simulink model "PV_&_LV_FEEDER_MODEL"  (R2024b)
settings: Solver=ode23s  StartTime=0.0  StopTime=2.4  RelTol=1e-3
libraries: spsFirstOrderFilterLib x54, spsSeriesRLCBranchLib x12, spsThreePhaseVIMeasurementLib x9, spsIGBTDiodeLib x7, slpidlib x5, spsThreePhaseDynamicLoadLib x4, spsDistributedParametersLineLib x4, spsPower3phInstantaneousLib x4, simulink x3, spsThreePhaseSourceLib x2, spsThreePhaseTransformerTwoWindingsLib x2, spsabctodq0Lib x2
(part 2 of 3)

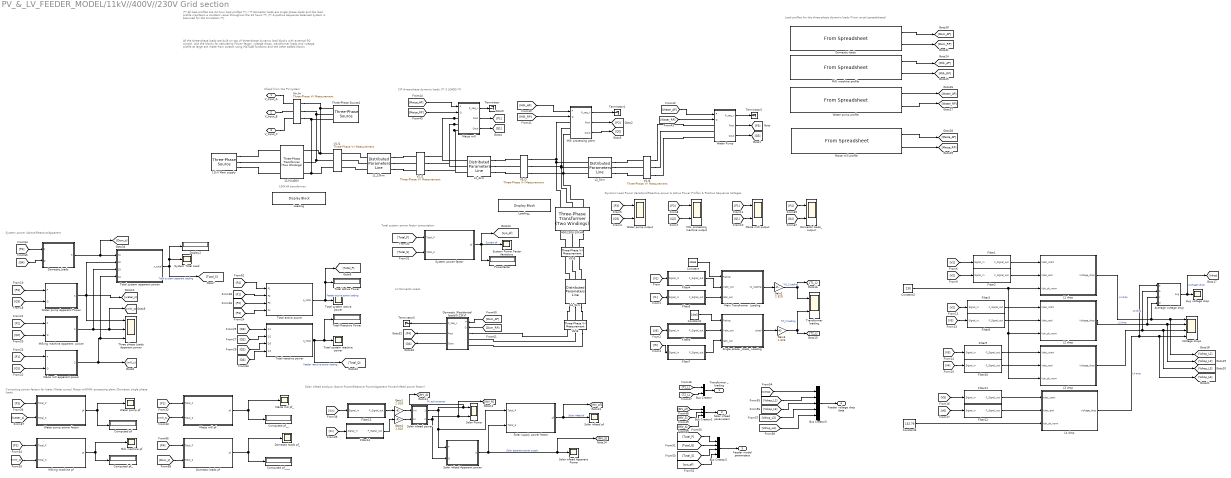
== system PV_&_LV_FEEDER_MODEL/11kV//400V//230V Grid section ==
  note: Load profiles for the three-phase dynamic loads (From excel spreadsheets)
  note: Total system power factor computation
  note: System power /Acitve/Reactive/Apparent
  note: 100kVA transformer
  note: Dynamic Load Power Variations(Reactive power & Active Power Profile) & Positive Sequence Voltages
  note: All the three-phase loads are built on top of three-phase dynamic load blocks with external PQ control.
      |
      | And the blocks for calculating Power factor, voltage drops, transfromer loads and voltage profile at large are made from scratch using MATLAB functions and the other added blocks
  note: Infeed from the PV system
  note: LV Domestic Loads
  note: CIP three-phase dynamic loads /** 3 LOADS **/
  note: /** All load profiles are 24 hour load profiles **/
      |
      | / ** Domestic loads are single phase loads and the load profile maintains a constant value throughout the 24 hours **/
      |
      | /** A postive sequence balanced system is assumed for the simulation **/
  note: Solar infeed analysis (Active Power/Reactive Power/Apparent Power/Infeed power factor)
  note: Computing power factors for loads /Water pump/ Maize mill/Milk processing plant /Domestic single phase loads
  11kV Main supply : spsThreePhaseSourceLib/Three-Phase Source  InternalConnection=Yg  VoltagePhases=off  Voltage=11e3  PhaseAngle=0  Voltage_phases=[25e3 25e3 25e3]/sqrt(3)  PhaseAngles_phases=[0 -120 +120]  Frequency=50  NonIdealSource=on  SpecifyImpedance=off  Resistance=0.8929  Inductance=16.58e-3  ShortCircuitLevel=100e6  BaseVoltage=25e3  XRratio=7  BusType=swing  Pref=10e3  Qref=0  Prefabc=[10e3, 10e3, 10e3]  Qrefabc=[0, 0, 0]  Qmin=-inf  Qmax=inf
  "11kV/400V " : spsThreePhaseTransformerTwoWindingsLib/Three-Phase Transformer (Two Windings)  Winding1Connection=Yg  Winding2Connection=Yg  CoreType=Three single-phase transformers  SetSaturation=off  Hysteresis=off  DataFile='hysteresis'  SetInitialFlux=off  Measurements=None  UNITS=pu  NominalPower=[ 100e3 , 50 ]  Winding1=[ 11e3 , 0.002 , 0.08 ]  Winding2=[ 400 , 0.002 , 0.08 ]  Rm=500  Lm=500  L0=0.5  Saturation=[ 0,0 ; 0.0024,1.2 ; 1.0,1.52 ]  InitialFluxes=[ 0.8 , -0.8 , 0.7 ]  BreakLoop=off  DiscreteSolver=Trapezoidal iterative  DataType=off  TransfoNumber=1
  "400/230V-10kVA " : spsThreePhaseTransformerTwoWindingsLib/Three-Phase Transformer (Two Windings)  Winding1Connection=Yg  Winding2Connection=Yg  CoreType=Three single-phase transformers  SetSaturation=off  Hysteresis=off  DataFile='hysteresis'  SetInitialFlux=off  Measurements=None  UNITS=pu  NominalPower=[ 10e3 , 50 ]  Winding1=[ 400 , 0.002 , 0.08 ]  Winding2=[ 230 , 0.002 , 0.08 ]  Rm=500  Lm=500  L0=0.5  Saturation=[ 0,0 ; 0.0024,1.2 ; 1.0,1.52 ]  InitialFluxes=[ 0.8 , -0.8 , 0.7 ]  BreakLoop=off  DiscreteSolver=Trapezoidal iterative  DataType=off  TransfoNumber=1
  Average voltage drop : MATLAB Function  TreatAsAtomicUnit=on
  Avg voltage drop : Scope
  Bus Creator : BusCreator  Inputs=2
  Bus Creator1 : BusCreator  Inputs=3
  Bus Creator2 : BusCreator  Inputs=4
  Bus Creator3 : BusCreator  Inputs=5
  Computed pf : Display
  Computed pf_ : Display
  Computed pf__ : Display
  Computed pf____ : Display
  Constant : Constant  Value=100e3
  Constant1 : Constant  Value=10e3
  Constant2 : Constant  Value=230
  Constant3 : Constant  Value=132.79
  Display2 : Display
  Domestic /Residential loads(0.23kV) : Subsystem
  Domestic loads : FromSpreadsheet  FileName=C:\Users\Baymax\Desktop\Mr.Usamah\Profiles\granular\h_pf\Domestic_loads.xlsx  SheetName=profile  Range=A2:C2002
  Domestic loads pf : MATLAB Function  TreatAsAtomicUnit=on
  Domestic loads pf_ : Scope
  Domestic loads_output : Scope  NumInputPorts=2
  Domestic_loads : MATLAB Function  TreatAsAtomicUnit=on
  Filter1 : Subsystem
  Filter10 : Subsystem
  Filter11 : Subsystem
  Filter12 : Subsystem
  Filter13 : Subsystem
  Filter14 : Subsystem
  Filter2 : Subsystem
  Filter3 : Subsystem
  Filter4 : Subsystem
  Filter5 : Subsystem
  Filter6 : Subsystem
  Filter7 : Subsystem
  Filter8 : Subsystem
  Filter9 : Subsystem
  Gain{1..4} (4 alike) : Gain  Gain=2.828
  L1 drop : Subsystem
  L1_10km : spsDistributedParametersLineLib/Distributed Parameters Line  Phases=3  Length=10  Frequency=50  Resistance=[0.01273 0.3864]  Inductance="[0.9337e-3  4.1264e-3]"  Capacitance=[12.74e-9 7.751e-9]  x1=[-5.7e-05 -1.52676771420257e-15 0 0;-5.6e-05 -1.49998510389932e-15 0 0;-5.5e-05 -1.47320234555348e-15 0 0;-5.4e-05 -1.44641944180839e-15 0 0;-5.3e-05 -1.41963639530743e-15 0 0;-5.2e-05 -1.39285320869397e-15 0 0;-5.1e-05 -1.36606988461142e-15 0 0;-5e-05 -1.33928642570317e-15 0 0;-4.9e-05 -1.31250283461264e-15 0 0;-4.8e-05 -1.28571911398329e-15 0 0;-4.7e-05 -1.25893526645854e-15 0 0;-4.6e-05 -1.23215129468186e-15 0 0;-4.5e-05 -1.20536720129673e-15 0 0;-4.4e-05 -1.17858298894662e-15 0 0;-4.3e-05 -1.15179866027504e-15 0 0;-4.2e-05 -1.12501421792548e-15 0 0;-4.1e-05 -1.09822966454148e-15 0 0;-4e-05 -1.07144500276655e-15 0 0;-3.9e-05 -1.04466023524424e-15 0 0;-3.8e-05 -1.01787536461809e-15 0 0;-3.7e-05 -9.91090393531678e-16 0 0;-3.6e-05 -9.64305324628563e-16 0 0;-3.5e-05 -9.37520160552329e-16 196.179007943669 -348.588291315468;-3.4e-05 -9.10734903946564e-16 196.288510502334 -348.526642661325;-3.3e-05 -8.83949557454868e-16 196.3979936881 -348.464959608981;-3.2e-05 -8.57164123720848e-16 196.507457490161 -348.403242164525;-3.1e-05 -8.30378605388121e-16 196.616901897713 -348.341490334047;-3e-05 -8.03593005100311e-16 196.726326899956 -348.279704123642;-2.9e-05 -7.76807325501051e-16 196.835732486088 -348.217883539409;-2.8e-05 -7.50021569233982e-16 196.945118645312 -348.156028587448;-2.7e-05 -7.23235738942752e-16 197.054485366832 -348.094139273865;-2.6e-05 -6.96449837271016e-16 197.163832639854 -348.032215604768;-2.5e-05 -6.69663866862436e-16 197.273160453586 -347.970257586268;-2.4e-05 -6.42877830360683e-16 197.382468797238 -347.90826522448;-2.3e-05 -6.16091730409431e-16 197.491757660021 -347.846238525524;-2.2e-05 -5.89305569652364e-16 197.601027031149 -347.78417749552;-2.1e-05 -5.62519350733168e-16 197.710276899837 -347.722082140594;-2e-05 -5.35733076295539e-16 197.819507255304 -347.659952466874;-1.9e-05 -5.08946748983174e-16 197.928718086768 -347.597788480492;-1.8e-05 -4.82160371439779e-16 198.03790938345 -347.535590187584;-1.7e-05 -4.55373946309064e-16 198.147081134575 -347.473357594289;-1.6e-05 -4.28587476234741e-16 198.256233329366 -347.411090706748;-1.5e-05 -4.01800963860531e-16 198.365365957052 -347.348789531107;-1.4e-05 -3.75014411830155e-16 198.474479006861 -347.286454073514;-1.3e-05 -3.48227822787341e-16 198.583572468024 -347.224084340123;-1.2e-05 -3.21441199375819e-16 198.692646329775 -347.161680337089;-1.1e-05 -2.94654544239322e-16 198.801700581347 -347.09924207057;-1e-05 -2.67867860021587e-16 198.910735211978 -347.03676954673;-9e-06 -2.41081149366355e-16 199.019750210907 -346.974262771734;-8e-06 -2.14294414917367e-16 199.128745567374 -346.911721751751;-7e-06 -1.87507659318368e-16 199.237721270622 -346.849146492953;-6e-06 -1.60720885213105e-16 199.346677309894 -346.786537001518;-5e-06 -1.33934095245327e-16 199.455613674439 -346.723893283623;-4e-06 -1.07147292058783e-16 199.564530353504 -346.661215345452;-3e-06 -8.03604782972257e-17 199.673427336339 -346.59850319319;-2e-06 -5.35736566044071e-17 199.782304612197 -346.535756833028;-1e-06 -2.67868296240806e-17 199.891162170332 -346.472976271158]  x2=[-5.7e-05 -2.62897177572208e-12 0 0;-5.6e-05 -2.62972765843218e-12 0 0;-5.5e-05 -2.63048328159856e-12 0 0;-5.4e-05 -2.63123864514666e-12 0 0;-5.3e-05 -2.63199374900191e-12 0 0;-5.2e-05 -2.63274859308979e-12 0 0;-5.1e-05 -2.6335031773358e-12 0 0;-5e-05 -2.63425750166547e-12 0 0;-4.9e-05 -2.63501156600435e-12 0 0;-4.8e-05 -2.63576537027801e-12 0 0;-4.7e-05 -2.63651891441206e-12 0 0;-4.6e-05 -2.63727219833213e-12 0 0;-4.5e-05 -2.63802522196386e-12 0 0;-4.4e-05 -2.63877798523294e-12 0 0;-4.3e-05 -2.63953048806508e-12 0 0;-4.2e-05 -2.640282730386e-12 0 0;-4.1e-05 -2.64103471212147e-12 0 0;-4e-05 -2.64178643319725e-12 0 0;-3.9e-05 -2.64253789353917e-12 0 0;-3.8e-05 -2.64328909307306e-12 0 0;-3.7e-05 -2.64404003172477e-12 0 0;-3.6e-05 -2.64479070942019e-12 0 0;-3.5e-05 -2.64554112608523e-12 132.127149459759 -329.646500354157;-3.4e-05 -2.64629128164583e-12 132.230307052903 -329.60328299373;-3.3e-05 -2.64704117602796e-12 132.33345159544 -329.560033102763;-3.2e-05 -2.64779080915759e-12 132.436583077188 -329.516750685525;-3.1e-05 -2.64854018096075e-12 132.539701487969 -329.473435746288;-3e-05 -2.64928929136347e-12 132.642806817607 -329.430088289326;-2.9e-05 -2.65003814029182e-12 132.745899055924 -329.386708318918;-2.8e-05 -2.65078672767189e-12 132.848978192746 -329.343295839345;-2.7e-05 -2.6515350534298e-12 132.9520442179 -329.299850854891;-2.6e-05 -2.65228311749169e-12 133.055097121213 -329.256373369846;-2.5e-05 -2.65303091978374e-12 133.158136892514 -329.212863388499;-2.4e-05 -2.65377846023213e-12 133.261163521634 -329.169320915145;-2.3e-05 -2.65452573876308e-12 133.364176998405 -329.125745954082;-2.2e-05 -2.65527275530285e-12 133.467177312659 -329.08213850961;-2.1e-05 -2.6560195097777e-12 133.570164454231 -329.038498586033;-2e-05 -2.65676600211394e-12 133.673138412956 -328.994826187658;-1.9e-05 -2.65751223223789e-12 133.776099178671 -328.951121318796;-1.8e-05 -2.65825820007589e-12 133.879046741214 -328.907383983759;-1.7e-05 -2.65900390555433e-12 133.981981090426 -328.863614186865;-1.6e-05 -2.6597493485996e-12 134.084902216146 -328.819811932434;-1.5e-05 -2.66049452913813e-12 134.187810108216 -328.775977224788;-1.4e-05 -2.66123944709639e-12 134.290704756481 -328.732110068254;-1.3e-05 -2.66198410240084e-12 134.393586150785 -328.688210467162;-1.2e-05 -2.66272849497799e-12 134.496454280973 -328.644278425844;-1.1e-05 -2.66347262475438e-12 134.599309136893 -328.600313948636;-1e-05 -2.66421649165655e-12 134.702150708395 -328.556317039877;-9e-06 -2.6649600956111e-12 134.804978985327 -328.51228770391;-8e-06 -2.66570343654463e-12 134.907793957541 -328.468225945079;-7e-06 -2.66644651438379e-12 135.010595614889 -328.424131767735;-6e-06 -2.66718932905522e-12 135.113383947226 -328.380005176228;-5e-06 -2.66793188048562e-12 135.216158944407 -328.335846174914;-4e-06 -2.66867416860169e-12 135.318920596287 -328.291654768151;-3e-06 -2.66941619333019e-12 135.421668892726 -328.247430960301;-2e-06 -2.67015795459787e-12 135.524403823582 -328.203174755729;-1e-06 -2.67089945233153e-12 135.627125378715 -328.158886158801]  x3=[-5.7e-05 1.17698290725369e-13 0 0;-5.6e-05 1.1762296132752e-13 0 0;-5.5e-05 1.1754762032075e-13 0 0;-5.4e-05 1.17472267712495e-13 0 0;-5.3e-05 1.17396903510192e-13 0 0;-5.2e-05 1.17321527721279e-13 0 0;-5.1e-05 1.17246140353195e-13 0 0;-5e-05 1.17170741413382e-13 0 0;-4.9e-05 1.17095330909279e-13 0 0;-4.8e-05 1.17019908848331e-13 0 0;-4.7e-05 1.16944475237981e-13 0 0;-4.6e-05 1.16869030085674e-13 0 0;-4.5e-05 1.16793573398857e-13 0 0;-4.4e-05 1.16718105184975e-13 0 0;-4.3e-05 1.16642625451479e-13 0 0;-4.2e-05 1.16567134205817e-13 0 0;-4.1e-05 1.1649163145544e-13 0 0;-4e-05 1.16416117207799e-13 0 0;-3.9e-05 1.16340591470349e-13 0 0;-3.8e-05 1.16265054250543e-13 0 0;-3.7e-05 1.16189505555836e-13 0 0;-3.6e-05 1.16113945393684e-13 0 0;-3.5e-05 1.16038373771546e-13 6.64607990253194 18.9464899277629;-3.4e-05 1.15962790696879e-13 6.63954583439883 18.948466711769;-3.3e-05 1.15887196177143e-13 6.63301111096882 18.9504416256364;-3.2e-05 1.158115902198e-13 6.62647573288685 18.9524146691702;-3.1e-05 1.15735972832311e-13 6.61993970079795 18.9543858421757;-3e-05 1.1566034402214e-13 6.6134030153472 18.9563551444583;-2.9e-05 1.1558470379675e-13 6.60686567717974 18.9583225758237;-2.8e-05 1.15509052163607e-13 6.60032768694077 18.9602881360776;-2.7e-05 1.15433389130178e-13 6.59378904527558 18.9622518250261;-2.6e-05 1.1535771470393e-13 6.58724975282951 18.9642136424754;-2.5e-05 1.15282028892332e-13 6.58070981024794 18.9661735882318;-2.4e-05 1.15206331702854e-13 6.57416921817636 18.968131662102;-2.3e-05 1.15130623142967e-13 6.56762797726028 18.9700878638926;-2.2e-05 1.15054903220143e-13 6.56108608814531 18.9720421934106;-2.1e-05 1.14979171941855e-13 6.55454355147711 18.9739946504631;-2e-05 1.14903429315578e-13 6.54800036790139 18.9759452348574;-1.9e-05 1.14827675348787e-13 6.54145653806395 18.977893946401;-1.8e-05 1.14751910048959e-13 6.53491206261062 18.9798407849015;-1.7e-05 1.14676133423572e-13 6.52836694218734 18.9817857501669;-1.6e-05 1.14600345480103e-13 6.52182117744007 18.9837288420051;-1.5e-05 1.14524546226035e-13 6.51527476901485 18.9856700602244;-1.4e-05 1.14448735668846e-13 6.5087277175578 18.9876094046332;-1.3e-05 1.1437291381602e-13 6.50218002371507 18.9895468750401;-1.2e-05 1.14297080675041e-13 6.4956316881329 18.9914824712538;-1.1e-05 1.14221236253391e-13 6.48908271145759 18.9934161930834;-1e-05 1.14145380558558e-13 6.48253309433549 18.9953480403379;-9e-06 1.14069513598027e-13 6.47598283741302 18.9972780128267;-8e-06 1.13993635379286e-13 6.46943194133667 18.9992061103594;-7e-06 1.13917745909825e-13 6.46288040675299 19.0011323327456;-6e-06 1.13841845197133e-13 6.45632823430858 19.0030566797952;-5e-06 1.13765933248701e-13 6.44977542465012 19.0049791513184;-4e-06 1.13690010072022e-13 6.44322197842435 19.0068997471252;-3e-06 1.13614075674589e-13 6.43666789627806 19.0088184670263;-2e-06 1.13538130063896e-13 6.43011317885812 19.0107353108322;-1e-06 1.13462173247438e-13 6.42355782681145 19.0126502783538]  x4=[-5.7e-05 -1.21011045818771e-13 0 0;-5.6e-05 -1.20939770771355e-13 0 0;-5.5e-05 -1.20868483787662e-13 0 0;-5.4e-05 -1.20797184874728e-13 0 0;-5.3e-05 -1.2072587403959e-13 0 0;-5.2e-05 -1.20654551289286e-13 0 0;-5.1e-05 -1.20583216630855e-13 0 0;-5e-05 -1.20511870071338e-13 0 0;-4.9e-05 -1.20440511617776e-13 0 0;-4.8e-05 -1.20369141277212e-13 0 0;-4.7e-05 -1.2029775905669e-13 0 0;-4.6e-05 -1.20226364963256e-13 0 0;-4.5e-05 -1.20154959003954e-13 0 0;-4.4e-05 -1.20083541185834e-13 0 0;-4.3e-05 -1.20012111515944e-13 0 0;-4.2e-05 -1.19940670001333e-13 0 0;-4.1e-05 -1.19869216649052e-13 0 0;-4e-05 -1.19797751466154e-13 0 0;-3.9e-05 -1.19726274459692e-13 0 0;-3.8e-05 -1.1965478563672e-13 0 0;-3.7e-05 -1.19583285004294e-13 0 0;-3.6e-05 -1.19511772569472e-13 0 0;-3.5e-05 -1.1944024833931e-13 -5.44733327904661 -21.4575907170846;-3.4e-05 -1.19368712320869e-13 -5.44001188573569 -21.4591845394917;-3.3e-05 -1.19297164521207e-13 -5.43268995551713 -21.4607762439623;-3.2e-05 -1.19225604947388e-13 -5.42536748911357 -21.4623658303391;-3.1e-05 -1.19154033606473e-13 -5.4180444872477 -21.4639532984654;-3e-05 -1.19082450505527e-13 -5.41072095064228 -21.4655386481844;-2.9e-05 -1.19010855651614e-13 -5.40339688002011 -21.4671218793397;-2.8e-05 -1.189392490518e-13 -5.39607227610405 -21.4687029917749;-2.7e-05 -1.18867630713153e-13 -5.38874713961701 -21.4702819853342;-2.6e-05 -1.18796000642742e-13 -5.38142147128195 -21.4718588598616;-2.5e-05 -1.18724358847635e-13 -5.37409527182188 -21.4734336152014;-2.4e-05 -1.18652705334903e-13 -5.36676854195987 -21.4750062511983;-2.3e-05 -1.18581040111619e-13 -5.35944128241904 -21.4765767676971;-2.2e-05 -1.18509363184856e-13 -5.35211349392256 -21.4781451645427;-2.1e-05 -1.18437674561687e-13 -5.34478517719366 -21.4797114415804;-2e-05 -1.18365974249189e-13 -5.33745633295561 -21.4812755986556;-1.9e-05 -1.18294262254437e-13 -5.33012696193174 -21.4828376356138;-1.8e-05 -1.1822253858451e-13 -5.32279706484543 -21.484397552301;-1.7e-05 -1.18150803246486e-13 -5.31546664242011 -21.4859553485632;-1.6e-05 -1.18079056247445e-13 -5.30813569537926 -21.4875110242466;-1.5e-05 -1.18007297594468e-13 -5.30080422444643 -21.4890645791976;-1.4e-05 -1.17935527294638e-13 -5.29347223034519 -21.490616013263;-1.3e-05 -1.17863745355039e-13 -5.28613971379918 -21.4921653262897;-1.2e-05 -1.17791951782754e-13 -5.27880667553211 -21.4937125181247;-1.1e-05 -1.17720146584869e-13 -5.2714731162677 -21.4952575886152;-1e-05 -1.17648329768472e-13 -5.26413903672975 -21.496800537609;-9e-06 -1.1757650134065e-13 -5.25680443764211 -21.4983413649535;-8e-06 -1.17504661308492e-13 -5.24946931972867 -21.4998800704969;-7e-06 -1.1743280967909e-13 -5.24213368371339 -21.5014166540871;-6e-06 -1.17360946459533e-13 -5.23479753032024 -21.5029511155726;-5e-06 -1.17289071656916e-13 -5.2274608602733 -21.5044834548019;-4e-06 -1.17217185278332e-13 -5.22012367429665 -21.5060136716238;-3e-06 -1.17145287330875e-13 -5.21278597311445 -21.5075417658872;-2e-06 -1.17073377821642e-13 -5.2054477574509 -21.5090677374414;-1e-06 -1.17001456757729e-13 -5.19810902803026 -21.5105915861357]  x5=5.65541566995743e-05  V1=ones(3,3)  V2=ones(3,3)  I1=ones(3,3)  I2=ones(3,3)  nHarmo=1  Measurements=None  Decoupling=off  VsMag0=0  VrMag0=0  VsAngle0=0  VrAngle0=0  IsMag0=0  IrMag0=0  IsAngle0=0  IrAngle0=0
      settings: LibrarySourceBlock=sps_lib/Power Grid Elements/Distributed Parameters Line
  L2 drop : Subsystem
  L2_3km : spsDistributedParametersLineLib/Distributed Parameters Line  Phases=3  Length=3  Frequency=50  Resistance=[0.01273 0.3864]  Inductance="[0.9337e-3  4.1264e-3]"  Capacitance=[12.74e-9 7.751e-9]  x1=[-1.7e-05 -2.65900390555433e-12 0 0;-1.6e-05 -2.6597493485996e-12 0 0;-1.5e-05 -2.66049452913813e-12 0 0;-1.4e-05 -2.66123944709639e-12 0 0;-1.3e-05 -2.66198410240084e-12 0 0;-1.2e-05 -2.66272849497799e-12 0 0;-1.1e-05 -2.66347262475438e-12 134.599309136893 -328.600313948636;-1e-05 -2.66421649165655e-12 134.702150708395 -328.556317039877;-9e-06 -2.6649600956111e-12 134.804978985327 -328.51228770391;-8e-06 -2.66570343654463e-12 134.907793957541 -328.468225945079;-7e-06 -2.66644651438379e-12 135.010595614889 -328.424131767735;-6e-06 -2.66718932905522e-12 135.113383947226 -328.380005176228;-5e-06 -2.66793188048562e-12 135.216158944407 -328.335846174914;-4e-06 -2.66867416860169e-12 135.318920596287 -328.291654768151;-3e-06 -2.66941619333019e-12 135.421668892726 -328.247430960301;-2e-06 -2.67015795459787e-12 135.524403823582 -328.203174755729;-1e-06 -2.67089945233153e-12 135.627125378715 -328.158886158801]  x2=[-1.7e-05 -1.06786625029648e-12 0 0;-1.6e-05 -1.06858231496139e-12 0 0;-1.5e-05 -1.06929827416146e-12 0 0;-1.4e-05 -1.07001412782602e-12 0 0;-1.3e-05 -1.07072987588442e-12 0 0;-1.2e-05 -1.07144551826601e-12 0 0;-1.1e-05 -1.07216105490018e-12 117.837536827924 -323.773646079117;-1e-05 -1.07287648571629e-12 117.938747506776 -323.73440678193;-9e-06 -1.07359181064373e-12 118.039946545541 -323.695135533439;-8e-06 -1.07430702961191e-12 118.14113393423 -323.655832337518;-7e-06 -1.07502214255024e-12 118.242309662856 -323.616497198048;-6e-06 -1.07573714938814e-12 118.343473721435 -323.57713011891;-5e-06 -1.07645205005503e-12 118.44462609998 -323.537731103989;-4e-06 -1.07716684448037e-12 118.54576678851 -323.498300157174;-3e-06 -1.0778815325936e-12 118.646895777042 -323.458837282357;-2e-06 -1.07859611432419e-12 118.748013055595 -323.419342483433;-1e-06 -1.07931058960162e-12 118.849118614188 -323.379815764299]  x3=[-1.7e-05 6.00604604613741e-14 0 0;-1.6e-05 6.01818414409508e-14 0 0;-1.5e-05 6.0303216480818e-14 0 0;-1.4e-05 6.04245855689962e-14 0 0;-1.3e-05 6.0545948693507e-14 0 0;-1.2e-05 6.06673058423722e-14 0 0;-1.1e-05 6.07886570036144e-14 5.56089804964976 16.1978590482491;-1e-05 6.09100021652566e-14 5.5552252459904 16.199505686642;-9e-06 6.10313413153226e-14 5.5495518940523 16.2011507262079;-8e-06 6.11526744418368e-14 5.54387799439538 16.2027941667843;-7e-06 6.12740015328239e-14 5.53820354757964 16.204436008209;-6e-06 6.13953225763096e-14 5.53252855416512 16.20607625032;-5e-06 6.15166375603198e-14 5.52685301471193 16.2077148929554;-4e-06 6.16379464728813e-14 5.52117692978021 16.2093519359535;-3e-06 6.17592493020214e-14 5.51550029993018 16.2109873791527;-2e-06 6.18805460357679e-14 5.50982312572209 16.2126212223915;-1e-06 6.20018366621494e-14 5.50414540771625 16.2142534655088]  x4=[-1.7e-05 -6.87075593118103e-14 0 0;-1.6e-05 -6.88423373437948e-14 0 0;-1.5e-05 -6.89771085813131e-14 0 0;-1.4e-05 -6.91118730110636e-14 0 0;-1.3e-05 -6.92466306197458e-14 0 0;-1.2e-05 -6.93813813940595e-14 0 0;-1.1e-05 -6.95161253207054e-14 -4.63242844236993 -18.6089754457082;-1e-05 -6.96508623863848e-14 -4.62600150068479 -18.6103158835768;-9e-06 -6.97855925777997e-14 -4.6195741024316 -18.6116544846809;-8e-06 -6.99203158816527e-14 -4.61314624824473 -18.6129912488883;-7e-06 -7.00550322846471e-14 -4.60671793875858 -18.6143261760672;-6e-06 -7.01897417734871e-14 -4.60028917460759 -18.6156592660857;-5e-06 -7.03244443348774e-14 -4.59385995642626 -18.6169905188123;-4e-06 -7.04591399555232e-14 -4.58743028484914 -18.6183199341155;-3e-06 -7.05938286221307e-14 -4.58100016051079 -18.6196475118643;-2e-06 -7.07285103214066e-14 -4.57456958404586 -18.6209732519275;-1e-06 -7.08631850400584e-14 -4.56813855608901 -18.6222971541744]  x5=1.69662470098723e-05  V1=ones(3,3)  V2=ones(3,3)  I1=ones(3,3)  I2=ones(3,3)  nHarmo=1  Measurements=None  Decoupling=off  VsMag0=0  VrMag0=0  VsAngle0=0  VrAngle0=0  IsMag0=0  IrMag0=0  IsAngle0=0  IrAngle0=0
      settings: LibrarySourceBlock=sps_lib/Power Grid Elements/Distributed Parameters Line
  L3 drop : Subsystem
  L3_5km : spsDistributedParametersLineLib/Distributed Parameters Line  Phases=3  Length=5  Frequency=50  Resistance=[0.01273 0.3864]  Inductance="[0.9337e-3  4.1264e-3]"  Capacitance=[12.74e-9 7.751e-9]  x1=[-2.9e-05 -1.05926527379479e-12 0 0;-2.8e-05 -1.05998259852241e-12 0 0;-2.7e-05 -1.06069981863395e-12 0 0;-2.6e-05 -1.06141693405861e-12 0 0;-2.5e-05 -1.06213394472562e-12 0 0;-2.4e-05 -1.06285085056421e-12 0 0;-2.3e-05 -1.06356765150363e-12 0 0;-2.2e-05 -1.06428434747313e-12 0 0;-2.1e-05 -1.06500093840198e-12 0 0;-2e-05 -1.06571742421944e-12 0 0;-1.9e-05 -1.06643380485482e-12 0 0;-1.8e-05 -1.06715008023739e-12 117.128736992729 -324.047426197968;-1.7e-05 -1.06786625029648e-12 117.230028872437 -324.008410668177;-1.6e-05 -1.06858231496139e-12 117.331309182004 -323.969363160038;-1.5e-05 -1.06929827416146e-12 117.432577911436 -323.930283677405;-1.4e-05 -1.07001412782602e-12 117.533835050737 -323.891172224135;-1.3e-05 -1.07072987588442e-12 117.635080589913 -323.852028804087;-1.2e-05 -1.07144551826601e-12 117.736314518973 -323.812853421126;-1.1e-05 -1.07216105490018e-12 117.837536827924 -323.773646079117;-1e-05 -1.07287648571629e-12 117.938747506776 -323.73440678193;-9e-06 -1.07359181064373e-12 118.039946545541 -323.695135533439;-8e-06 -1.07430702961191e-12 118.14113393423 -323.655832337518;-7e-06 -1.07502214255024e-12 118.242309662856 -323.616497198048;-6e-06 -1.07573714938814e-12 118.343473721435 -323.57713011891;-5e-06 -1.07645205005503e-12 118.44462609998 -323.537731103989;-4e-06 -1.07716684448037e-12 118.54576678851 -323.498300157174;-3e-06 -1.0778815325936e-12 118.646895777042 -323.458837282357;-2e-06 -1.07859611432419e-12 118.748013055595 -323.419342483433;-1e-06 -1.07931058960162e-12 118.849118614188 -323.379815764299]  x2=[-2.9e-05 -2.11828092607484e-13 0 0;-2.8e-05 -2.12364447289422e-13 0 0;-2.7e-05 -2.1290078101183e-13 0 0;-2.6e-05 -2.13437093721773e-13 0 0;-2.5e-05 -2.1397338536632e-13 0 0;-2.4e-05 -2.1450965589254e-13 0 0;-2.3e-05 -2.15045905247506e-13 0 0;-2.2e-05 -2.15582133378292e-13 0 0;-2.1e-05 -2.16118340231974e-13 0 0;-2e-05 -2.16654525755631e-13 0 0;-1.9e-05 -2.17190689896344e-13 0 0;-1.8e-05 -2.17726832601195e-13 115.046538856704 -323.438678688607;-1.7e-05 -2.18262953817269e-13 115.147639586685 -323.400317298682;-1.6e-05 -2.18799053491654e-13 115.24872895205 -323.361923990425;-1.5e-05 -2.19335131571437e-13 115.349806942821 -323.323498767626;-1.4e-05 -2.19871188003711e-13 115.450873549023 -323.285041634077;-1.3e-05 -2.20407222735568e-13 115.551928760681 -323.246552593573;-1.2e-05 -2.20943235714105e-13 115.65297256782 -323.208031649914;-1.1e-05 -2.21479226886419e-13 115.754004960468 -323.169478806901;-1e-05 -2.22015196199609e-13 115.855025928654 -323.130894068339;-9e-06 -2.22551143600778e-13 115.956035462408 -323.092277438037;-8e-06 -2.2308706903703e-13 116.05703355176 -323.053628919805;-7e-06 -2.2362297245547e-13 116.158020186741 -323.014948517458;-6e-06 -2.24158853803209e-13 116.258995357386 -322.976236234814;-5e-06 -2.24694713027355e-13 116.359959053728 -322.937492075693;-4e-06 -2.25230550075022e-13 116.460911265802 -322.89871604392;-3e-06 -2.25766364893325e-13 116.561851983645 -322.859908143321;-2e-06 -2.26302157429381e-13 116.662781197295 -322.821068377726;-1e-06 -2.26837927630309e-13 116.763698896789 -322.78219675097]  x3=[-2.9e-05 -5.04825140254783e-14 0 0;-2.8e-05 -5.04388697117978e-14 0 0;-2.7e-05 -5.03952204200004e-14 0 0;-2.6e-05 -5.03515661543942e-14 0 0;-2.5e-05 -5.03079069192876e-14 0 0;-2.4e-05 -5.02642427189897e-14 0 0;-2.3e-05 -5.02205735578099e-14 0 0;-2.2e-05 -5.01768994400582e-14 0 0;-2.1e-05 -5.01332203700451e-14 0 0;-2e-05 -5.00895363520815e-14 0 0;-1.9e-05 -5.00458473904788e-14 0 0;-1.8e-05 -5.0002153489549e-14 0.782117828247901 0.236754840781964;-1.7e-05 -4.99584546536046e-14 0.782041502373816 0.23700866271578;-1.6e-05 -4.99147508869583e-14 0.781965099315328 0.237262461257778;-1.5e-05 -4.98710421939236e-14 0.781888619079979 0.237516236382911;-1.4e-05 -4.98273285788144e-14 0.781812061675318 0.23776998806613;-1.3e-05 -4.9783610045945e-14 0.781735427108899 0.238023716282393;-1.2e-05 -4.97398865996303e-14 0.781658715388287 0.238277421006656;-1.1e-05 -4.96961582441856e-14 0.781581926521053 0.238531102213881;-1e-05 -4.96524249839267e-14 0.781505060514775 0.23878475987903;-9e-06 -4.96086868231699e-14 0.781428117377039 0.239038393977068;-8e-06 -4.95649437662321e-14 0.781351097115441 0.239292004482963;-7e-06 -4.95211958174304e-14 0.781273999737581 0.239545591371683;-6e-06 -4.94774429810826e-14 0.781196825251068 0.239799154618201;-5e-06 -4.9433685261507e-14 0.78111957366352 0.240052694197492;-4e-06 -4.93899226630222e-14 0.78104224498256 0.240306210084531;-3e-06 -4.93461551899475e-14 0.780964839215822 0.240559702254299;-2e-06 -4.93023828466025e-14 0.780887356370944 0.240813170681775;-1e-06 -4.92586056373074e-14 0.780809796455574 0.241066615341945]  x4=[-2.9e-05 1.74202541006753e-14 0 0;-2.8e-05 1.73777795175095e-14 0 0;-2.7e-05 1.73353032192255e-14 0 0;-2.6e-05 1.72928252100157e-14 0 0;-2.5e-05 1.72503454940725e-14 0 0;-2.4e-05 1.72078640755885e-14 0 0;-2.3e-05 1.71653809587563e-14 0 0;-2.2e-05 1.7122896147769e-14 0 0;-2.1e-05 1.70804096468196e-14 0 0;-2e-05 1.70379214601013e-14 0 0;-1.9e-05 1.69954315918076e-14 0 0;-1.8e-05 1.69529400461321e-14 0.0689092844043278 -2.63052263321587;-1.7e-05 1.69104468272684e-14 0.0697338195339048 -2.63049272063614;-1.6e-05 1.68679519394105e-14 0.0705583477810297 -2.63046254843718;-1.5e-05 1.68254553867526e-14 0.0713828690643249 -2.63043211662197;-1.4e-05 1.67829571734888e-14 0.0722073833024133 -2.63040142519353;-1.3e-05 1.67404573038135e-14 0.0730318904139188 -2.63037047415487;-1.2e-05 1.66979557819213e-14 0.0738563903174656 -2.63033926350905;-1.1e-05 1.66554526120069e-14 0.0746808829316789 -2.63030779325915;-1e-05 1.66129477982653e-14 0.0755053681751846 -2.63027606340829;-9e-06 1.65704413448914e-14 0.0763298459666092 -2.63024407395958;-8e-06 1.65279332560806e-14 0.0771543162245801 -2.63021182491619;-7e-06 1.64854235360281e-14 0.0779787788677252 -2.6301793162813;-6e-06 1.64429121889296e-14 0.0788032338146734 -2.63014654805812;-5e-06 1.64003992189807e-14 0.0796276809840542 -2.63011352024989;-4e-06 1.63578846303773e-14 0.080452120294498 -2.63008023285985;-3e-06 1.63153684273154e-14 0.0812765516646358 -2.6300466858913;-2e-06 1.62728506139912e-14 0.0821009750130995 -2.63001287934755;-1e-06 1.6230331194601e-14 0.082925390258522 -2.62997881323194]  x5=2.82770783497871e-05  V1=ones(3,3)  V2=ones(3,3)  I1=ones(3,3)  I2=ones(3,3)  nHarmo=1  Measurements=None  Decoupling=off  VsMag0=0  VrMag0=0  VsAngle0=0  VrAngle0=0  IsMag0=0  IrMag0=0  IsAngle0=0  IrAngle0=0
      settings: LibrarySourceBlock=sps_lib/Power Grid Elements/Distributed Parameters Line
  L4 drop : Subsystem
  L4_5km : spsDistributedParametersLineLib/Distributed Parameters Line  Phases=3  Length=5  Frequency=50  Resistance=[0.01273 0.3864]  Inductance="[0.9337e-3  4.1264e-3]"  Capacitance=[12.74e-9 7.751e-9]  x1=[-2.9e-05 -8.0244010455671e-13 0 0;-2.8e-05 -8.01232439735496e-13 0 0;-2.7e-05 -8.0002469583581e-13 0 0;-2.6e-05 -7.98816872976853e-13 0 0;-2.5e-05 -7.97608971277831e-13 0 0;-2.4e-05 -7.96400990857959e-13 0 0;-2.3e-05 -7.95192931836461e-13 0 0;-2.2e-05 -7.93984794332567e-13 0 0;-2.1e-05 -7.92776578465515e-13 0 0;-2e-05 -7.91568284354552e-13 0 0;-1.9e-05 -7.90359912118932e-13 0 0;-1.8e-05 -7.89151461877915e-13 191.402487501905 38.5255314534738;-1.7e-05 -7.87942933750772e-13 191.412510896127 38.4647451318447;-1.6e-05 -7.86734327856778e-13 191.422515398692 38.4039550138975;-1.5e-05 -7.8552564431522e-13 191.432501008612 38.3431611056318;-1.4e-05 -7.84316883245388e-13 191.442467724902 38.2823634130479;-1.3e-05 -7.83108044766584e-13 191.452415546577 38.2215619421462;-1.2e-05 -7.81899128998114e-13 191.462344472657 38.1607566989275;-1.1e-05 -7.80690136059294e-13 191.472254502161 38.0999476893931;-1e-05 -7.79481066069447e-13 191.482145634111 38.0391349195447;-9e-06 -7.78271919147902e-13 191.492017867531 37.9783183953842;-8e-06 -7.77062695413999e-13 191.501871201446 37.9174981229139;-7e-06 -7.75853394987082e-13 191.511705634884 37.8566741081366;-6e-06 -7.74644017986505e-13 191.521521166875 37.7958463570553;-5e-06 -7.73434564531629e-13 191.53131779645 37.7350148756736;-4e-06 -7.72225034741821e-13 191.541095522641 37.6741796699951;-3e-06 -7.71015428736458e-13 191.550854344484 37.6133407460243;-2e-06 -7.69805746634924e-13 191.560594261016 37.5524981097655;-1e-06 -7.68595988556607e-13 191.570315271275 37.4916517672238]  x2=[-2.9e-05 -1.00023420414095e-12 0 0;-2.8e-05 -9.98821721480896e-13 0 0;-2.7e-05 -9.97409140241095e-13 0 0;-2.6e-05 -9.95996460560958e-13 0 0;-2.5e-05 -9.94583682579912e-13 0 0;-2.4e-05 -9.93170806437392e-13 0 0;-2.3e-05 -9.91757832272842e-13 0 0;-2.2e-05 -9.90344760225719e-13 0 0;-2.1e-05 -9.88931590435486e-13 0 0;-2e-05 -9.87518323041619e-13 0 0;-1.9e-05 -9.861049581836e-13 0 0;-1.8e-05 -9.84691496000924e-13 185.126767721522 44.7887696095556;-1.7e-05 -9.83277936633094e-13 185.137313955322 44.7295092762869;-1.6e-05 -9.81864280219622e-13 185.147841916802 44.6702445283925;-1.5e-05 -9.8045052690003e-13 185.158351604922 44.6109753717218;-1.4e-05 -9.79036676813851e-13 185.168843018646 44.5517018121243;-1.3e-05 -9.77622730100626e-13 185.179316156938 44.4924238554502;-1.2e-05 -9.76208686899905e-13 185.189771018764 44.4331415075498;-1.1e-05 -9.7479454735125e-13 185.200207603092 44.3738547742743;-1e-05 -9.7338031159423e-13 185.210625908892 44.3145636614748;-9e-06 -9.71965979768425e-13 185.221025935137 44.2552681750032;-8e-06 -9.70551552013423e-13 185.231407680799 44.1959683207118;-7e-06 -9.69137028468824e-13 185.241771144854 44.1366641044531;-6e-06 -9.67722409274234e-13 185.25211632628 44.0773555320804;-5e-06 -9.66307694569272e-13 185.262443224054 44.0180426094471;-4e-06 -9.64892884493564e-13 185.272751837159 43.9587253424071;-3e-06 -9.63477979186746e-13 185.283042164576 43.8994037368149;-2e-06 -9.62062978788463e-13 185.293314205289 43.8400777985252;-1e-06 -9.60647883438372e-13 185.303567958286 43.7807475333934]  x3=[-2.9e-05 -1.10655129817855e-13 0 0;-2.8e-05 -1.10655232077586e-13 0 0;-2.7e-05 -1.10655323416083e-13 0 0;-2.6e-05 -1.10655403833337e-13 0 0;-2.5e-05 -1.10655473329342e-13 0 0;-2.4e-05 -1.10655531904088e-13 0 0;-2.3e-05 -1.10655579557572e-13 0 0;-2.2e-05 -1.10655616289788e-13 0 0;-2.1e-05 -1.10655642100732e-13 0 0;-2e-05 -1.10655656990402e-13 0 0;-1.9e-05 -1.10655660958797e-13 0 0;-1.8e-05 -1.10655654005916e-13 -0.61055160802397 -2.97677042352867;-1.7e-05 -1.10655636131759e-13 -0.611840082940119 -2.9756106500902;-1.6e-05 -1.1065560733633e-13 -0.613128497470073 -2.97445058297072;-1.5e-05 -1.10655567619629e-13 -0.614416851486671 -2.97329022228475;-1.4e-05 -1.10655516981662e-13 -0.615705144862756 -2.97212956814679;-1.3e-05 -1.10655455422433e-13 -0.61699337747118 -2.97096862067141;-1.2e-05 -1.10655382941949e-13 -0.618281549184799 -2.96980737997318;-1.1e-05 -1.10655299540216e-13 -0.619569659876475 -2.96864584616671;-1e-05 -1.10655205217243e-13 -0.620857709419077 -2.96748401936664;-9e-06 -1.10655099973039e-13 -0.62214569768548 -2.96632189968764;-8e-06 -1.10654983807614e-13 -0.623433624548565 -2.96515948724441;-7e-06 -1.10654856720981e-13 -0.624721489881217 -2.96399678215166;-6e-06 -1.10654718713151e-13 -0.626009293556331 -2.96283378452417;-5e-06 -1.10654569784138e-13 -0.627297035446803 -2.9616704944767;-4e-06 -1.10654409933956e-13 -0.628584715425541 -2.96050691212407;-3e-06 -1.10654239162623e-13 -0.629872333365455 -2.95934303758113;-2e-06 -1.10654057470154e-13 -0.631159889139461 -2.95817887096273;-1e-06 -1.10653864856567e-13 -0.632447382620484 -2.95701441238379]  x4=[-2.9e-05 9.82072951349193e-14 0 0;-2.8e-05 9.82084073994252e-14 0 0;-2.7e-05 9.82095099711498e-14 0 0;-2.6e-05 9.82106028499844e-14 0 0;-2.5e-05 9.8211686035821e-14 0 0;-2.4e-05 9.82127595285529e-14 0 0;-2.3e-05 9.8213823328074e-14 0 0;-2.2e-05 9.82148774342794e-14 0 0;-2.1e-05 9.8215921847065e-14 0 0;-2e-05 9.82169565663277e-14 0 0;-1.9e-05 9.82179815919654e-14 0 0;-1.8e-05 9.8218996923877e-14 2.00049900265719 3.28829086762253;-1.7e-05 9.82200025619622e-14 2.00186462911222 3.2866879978948;-1.6e-05 9.82209985061218e-14 2.00323005799112 3.28508480378396;-1.5e-05 9.82219847562575e-14 2.00459528915915 3.28348128544825;-1.4e-05 9.82229613122719e-14 2.00596032248155 3.28187744304593;-1.3e-05 9.82239281740687e-14 2.00732515782361 3.2802732767353;-1.2e-05 9.82248853415524e-14 2.00868979505062 3.27866878667467;-1.1e-05 9.82258328146286e-14 2.01005423402789 3.2770639730224;-1e-05 9.82267705932038e-14 2.01141847462076 3.27545883593689;-9e-06 9.82276986771854e-14 2.01278251669459 3.27385337557655;-8e-06 9.82286170664818e-14 2.01414636011474 3.27224759209984;-7e-06 9.82295257610023e-14 2.01551000474662 3.27064148566523;-6e-06 9.82304247606574e-14 2.01687345045564 3.26903505643126;-5e-06 9.82313140653582e-14 2.01823669710723 3.26742830455646;-4e-06 9.82321936750169e-14 2.01959974456684 3.26582123019941;-3e-06 9.82330635895469e-14 2.02096259269995 3.26421383351873;-2e-06 9.82339238088621e-14 2.02232524137205 3.26260611467306;-1e-06 9.82347743328778e-14 2.02368769044865 3.26099807382107]  x5=2.82770783497871e-05  V1=ones(3,3)  V2=ones(3,3)  I1=ones(3,3)  I2=ones(3,3)  nHarmo=1  Measurements=None  Decoupling=off  VsMag0=0  VrMag0=0  VsAngle0=0  VrAngle0=0  IsMag0=0  IrMag0=0  IsAngle0=0  IrAngle0=0
      settings: LibrarySourceBlock=sps_lib/Power Grid Elements/Distributed Parameters Line
  Loading : DisplayBlock  LabelPosition=Hide  Transparency=1
  Loading_ : DisplayBlock  LabelPosition=Hide  Transparency=1
  Main Transfromer  Loading : Subsystem
  Maize mill : Subsystem
  Maize mill apparent power : MATLAB Function  TreatAsAtomicUnit=on
  Maize mill pf_ : Scope
  Maize mill profile : FromSpreadsheet  FileName=C:\Users\Baymax\Desktop\Mr.Usamah\Profiles\granular\h_pf\interpolated_maize_mill_hpf_profile.xlsx  SheetName=profile  Range=A3:C2002
  Maize milll output : Scope  NumInputPorts=2
  Miaze mill pf : MATLAB Function  TreatAsAtomicUnit=on
  Milk machine pf : Scope
  Milk machine profile : FromSpreadsheet  FileName=C:\Users\Baymax\Desktop\Mr.Usamah\Profiles\granular\h_pf\interpolated_milk_processing_plant_hpf_profile.xlsx  SheetName=profile  Range=A2:C2002
  Milk processing machine output : Scope  NumInputPorts=2
  Milk processing plant : Subsystem
  Milking machine apparent  power : MATLAB Function  TreatAsAtomicUnit=on
  Milking machine pf : MATLAB Function  TreatAsAtomicUnit=on
  Powerfactor : Display
  Single phase _loads_ Loading : Subsystem
  Solar Power : Scope  NumInputPorts=2
  Solar infeed Apparent Power : Scope
  Solar infeed Apparent power : MATLAB Function  TreatAsAtomicUnit=on
  Solar infeed pf : Scope
  Solar infeed power : Subsystem
  Solar supply power factor : MATLAB Function  TreatAsAtomicUnit=on
  System Power Factor Variations : Scope
  System Total Load : Scope
  System power factor : MATLAB Function  TreatAsAtomicUnit=on
  Terminator{,1..3} (4 alike) : Terminator
  Three phase Loads Apparent power : Scope  NumInputPorts=3
  Three-Phase Source1 : spsThreePhaseSourceLib/Three-Phase Source  InternalConnection=Yg  VoltagePhases=off  Voltage=400  PhaseAngle=0  Voltage_phases=[25e3 25e3 25e3]/sqrt(3)  PhaseAngles_phases=[0 -120 +120]  Frequency=50  NonIdealSource=off  SpecifyImpedance=off  Resistance=1e-6  Inductance=1e-6  ShortCircuitLevel=100e6  BaseVoltage=400  XRratio=7  BusType=swing  Pref=0  Qref=0  Prefabc=[10e3, 10e3, 10e3]  Qrefabc=[0, 0, 0]  Qmin=-inf  Qmax=inf
  Total Active Power : Display
  Total Reactive Power : Display
  Total active power : MATLAB Function  TreatAsAtomicUnit=on
  Total reactive power : MATLAB Function  TreatAsAtomicUnit=on
  Total system active power : Scope
  Total system apparent power : MATLAB Function  TreatAsAtomicUnit=on
  Total system reactive power : Scope
  Transformer loading : Scope  NumInputPorts=2
  V1,I1 : spsThreePhaseVIMeasurementLib/Three-Phase V-I Measurement  VoltageMeasurement=phase-to-ground  SetLabelV=on  LabelV=V1  Vpu=off  VpuLL=off  CurrentMeasurement=yes  SetLabelI=on  LabelI=I1  Ipu=off  Pbase=100e6  Vbase=500e3  OutputType=Complex  PhasorSimulation=off  PSBequivalent=0
  V2,I2 : spsThreePhaseVIMeasurementLib/Three-Phase V-I Measurement  VoltageMeasurement=phase-to-ground  SetLabelV=on  LabelV=V2  Vpu=off  VpuLL=off  CurrentMeasurement=yes  SetLabelI=on  LabelI=I2  Ipu=off  Pbase=100e6  Vbase=500e3  OutputType=Complex  PhasorSimulation=off  PSBequivalent=0
  V3,I3 : spsThreePhaseVIMeasurementLib/Three-Phase V-I Measurement  VoltageMeasurement=phase-to-ground  SetLabelV=on  LabelV=V3  Vpu=off  VpuLL=off  CurrentMeasurement=yes  SetLabelI=on  LabelI=I3  Ipu=off  Pbase=100e6  Vbase=500e3  OutputType=Complex  PhasorSimulation=off  PSBequivalent=0
  V4,I4 : spsThreePhaseVIMeasurementLib/Three-Phase V-I Measurement  VoltageMeasurement=phase-to-ground  SetLabelV=on  LabelV=V4  Vpu=off  VpuLL=off  CurrentMeasurement=yes  SetLabelI=on  LabelI=I4  Ipu=off  Pbase=100e6  Vbase=500e3  OutputType=Complex  PhasorSimulation=off  PSBequivalent=0
  V5,I5 : spsThreePhaseVIMeasurementLib/Three-Phase V-I Measurement  VoltageMeasurement=phase-to-ground  SetLabelV=on  LabelV=V5  Vpu=off  VpuLL=off  CurrentMeasurement=yes  SetLabelI=on  LabelI=I5  Ipu=off  Pbase=100e6  Vbase=500e3  OutputType=Complex  PhasorSimulation=off  PSBequivalent=0
  V6,I6 : spsThreePhaseVIMeasurementLib/Three-Phase V-I Measurement  VoltageMeasurement=phase-to-ground  SetLabelV=on  LabelV=V6  Vpu=off  VpuLL=off  CurrentMeasurement=yes  SetLabelI=on  LabelI=I6  Ipu=off  Pbase=100e6  Vbase=500e3  OutputType=Complex  PhasorSimulation=off  PSBequivalent=0
  Vin,Iin : spsThreePhaseVIMeasurementLib/Three-Phase V-I Measurement  VoltageMeasurement=phase-to-ground  SetLabelV=on  LabelV=Vin  Vpu=off  VpuLL=off  CurrentMeasurement=yes  SetLabelI=on  LabelI=Iin  Ipu=off  Pbase=100e6  Vbase=500e3  OutputType=Complex  PhasorSimulation=off  PSBequivalent=0
  Volltage drops : Scope  NumInputPorts=4
  Water Pump : Subsystem
  Water pump Apparent Power : MATLAB Function  TreatAsAtomicUnit=on
  Water pump output : Scope  NumInputPorts=2
  Water pump pf : Scope
  Water pump power factor : MATLAB Function  TreatAsAtomicUnit=on
  Water pump profile : FromSpreadsheet  FileName=C:\Users\Baymax\Desktop\Mr.Usamah\Profiles\granular\h_pf\interpolated_water_pump_hpf_profile.xlsx  SheetName=profile  Range=A2:C2002
  V_Input_A : PMIOPort  Side=Left
  V_Input_B : PMIOPort  Port=2  Side=Left
  V_Input_C : PMIOPort  Port=3  Side=Left
  Transformer _loading : Outport
  Solar infeed parameters : Outport  Port=2
  Feeder model parameters : Outport  Port=3
  Feeder voltage drop data : Outport  Port=4
  wires:
  Water pump Apparent Power/1(S) -> Three phase Loads Apparent power/1, [water_s], Total system apparent power/2(S2)
  [Q3] -> Water pump Apparent Power/2(Q)
  Filter4/1(F_Signal_out) -> Main Transfromer  Loading/2(Vabc_out)
  Maize mill apparent power/1(S) -> Total system apparent power/4(S4), Three phase Loads Apparent power/3, [mill_s]
  Filter2/1(F_Signal_out) -> L1 drop/2(Vabc_end)
  Constant2/1 -> L1 drop/3(Vph_ph_norm), L2 drop/3(Vph_ph_norm), L3 drop/3(Vph_ph_norm)
  [P3] -> Total active power/4(P4)
  [milk_s] -> Milking machine pf/2(Total_S)
  [I5] -> Filter7/1(Signal_in)
  [V1] -> Filter1/1(Signal_in)
  Total active power/1(p_total) -> [Total_P], Total Active Power/1, Total system active power/1  "Feeder active power loading"
  L2 drop/1(Voltage_drop) -> Average voltage drop/3(c), [Vdrop_L2], Volltage drops/2  "L2 drop"
  Milk processing plant/1(P_seq_v) -> Terminator1/1
  [V4] -> Filter10/1(Signal_in)
  Maize mill/1(P_seq_v) -> Terminator/1
  [P4] -> Total active power/1(P1)
  [P3] -> Water pump output/1
  Main Transfromer  Loading/1(t1_loading) -> Gain2/1
  Gain2/1 -> Transformer loading/1, [T1_L]  "Trf_1 loading"
  Average voltage drop/1(avg) -> [Vdrop], Avg voltage drop/1  "Average vdrop"
  [P1] -> Maize milll output/1
  [P3] -> Water pump Apparent Power/1(P)
  Filter5/1(F_Signal_out) -> Main Transfromer  Loading/3(Iabc_out)
  Filter9/1(F_Signal_out) -> L3 drop/1(Vabc_start)
  [Q1] -> Maize mill apparent power/2(Q)
  Domestic loads pf/1(pf) -> Domestic loads pf_/1, Computed pf____/1
  [V1] -> Filter4/1(Signal_in)
  Milk processing plant/3(Qout) -> [Q2]
  Water pump power factor/1(pf) -> Water pump pf/1, Computed pf/1
  Gain4/1 -> Solar infeed power/2(Iin)
  [Q3] -> Total reactive power/1(Q1)
  [Q4] -> Total reactive power/4(Q4)
  [mill_s] -> Miaze mill pf/2(Total_S)
  Constant1/1 -> Single phase _loads_ Loading/1(Rating)
  [P1] -> Miaze mill pf/1(Total_P)
  L4 drop/1(Voltage_drop) -> Average voltage drop/1(a), [Vdrop_L4], Volltage drops/4  "L4 drop"
  [Q2] -> Total reactive power/2(Q2)
  Constant/1 -> Main Transfromer  Loading/1(Rating)
  [V6] -> Filter12/1(Signal_in)
  [P2] -> Total active power/3(P3)
  [P1] -> Maize mill apparent power/1(P)
  Filter10/1(F_Signal_out) -> L3 drop/2(Vabc_end)
  System power factor/1(pf) -> [sys_pf], System Power Factor Variations/1, Powerfactor/1  "System pf"
  [V5] -> Filter11/1(Signal_in)
  Filter3/1(F_Signal_out) -> L2 drop/1(Vabc_start)
  Gain3/1 -> Transformer loading/2, [T2_L]  "Trf_2 loading"
  Milking machine pf/1(pf) -> Milk machine pf/1, Computed pf_/1
  L3 drop/1(Voltage_drop) -> Average voltage drop/2(b), [Vdrop_L3], Volltage drops/3  "L3 drop"
  [P1] -> Total active power/2(P2)
  Single phase _loads_ Loading/1(pload) -> Gain3/1
  Domestic_loads/1(S) -> [Dom_s], Total system apparent power/1(S1)
  [Q1] -> Maize milll output/2
  Filter12/1(F_Signal_out) -> L4 drop/2(Vabc_end)
  Solar infeed power/1(Inv_A) -> [INV_A], Solar Power/1, Solar supply power factor/1(Total_P), Solar infeed Apparent power/1(P)  "PV active power"
  [P2] -> Milking machine pf/1(Total_P)
  Miaze mill pf/1(pf) -> Maize mill pf_/1, Computed pf__/1
  Filter8/1(F_Signal_out) -> L2 drop/2(Vabc_end)
  Solar infeed power/2(Inv_R) -> [INV_R], Solar Power/2, Solar infeed Apparent power/2(Q)
  [Q2] -> Milking machine apparent  power/2(Q)
  Filter6/1(F_Signal_out) -> Single phase _loads_ Loading/2(Vabc_out)
  [Iin] -> Filter14/1(Signal_in)
  Total system apparent power/1(s_total) -> [Total_S], Display2/1, System Total Load/1  "Total system apparent loading"
  Total reactive power/1(q_total) -> Total Reactive Power/1, Total system reactive power/1, [Total_Q]  "Feeder reactive power loading"
  [V2] -> Filter3/1(Signal_in)
  Water Pump/3(Qout) -> [Q3]
  Gain1/1 -> Solar infeed power/1(Vin)
  Constant3/1 -> L4 drop/3(Vph_ph_norm)
  L1 drop/1(Voltage_drop) -> Average voltage drop/4(d), [Vdrop_L1], Volltage drops/1  "L1 drop"
  [V2] -> Filter2/1(Signal_in)
  [Q1] -> Total reactive power/3(Q3)
  [Water_RP] -> Water Pump/2(Q)
  [Maize_RP] -> Maize mill/2(Q)
  Milk machine profile/1 -> [Milk_AP]
  [Maize_AP] -> Maize mill/1(P)
  Maize mill profile/2 -> [Maize_RP]
  [I1] -> Filter5/1(Signal_in)
  Milking machine apparent  power/1(S) -> [milk_s], Three phase Loads Apparent power/2, Total system apparent power/3(S3)
  Water pump profile/1 -> [Water_AP]
  Filter1/1(F_Signal_out) -> L1 drop/1(Vabc_start)
  Water Pump/2(Pout) -> [P3]
  [P4] -> Domestic loads pf/1(Total_P)
  [Total_P] -> System power factor/1(Total_P)
  Solar infeed Apparent power/1(S) -> [INV_S], Solar infeed Apparent Power/1, Solar supply power factor/2(Total_S)  "Solar apparent power supply"
  Maize mill/2(Pout) -> [P1]
  [Total_S] -> System power factor/2(Total_S)
  Filter13/1(F_Signal_out) -> Gain1/1
  Milk processing plant/2(Pout) -> [P2]
  [Dom_s] -> Domestic loads pf/2(Total_S)
  [P2] -> Milk processing machine output/1
  Water Pump/1(P_seq_v) -> Terminator2/1
  [V5] -> Filter6/1(Signal_in)
  [Vin] -> Filter13/1(Signal_in)
  Filter14/1(F_Signal_out) -> Gain4/1
  [P2] -> Milking machine apparent  power/1(P)
  [Q2] -> Milk processing machine output/2
  Maize mill/3(Qout) -> [Q1]
  Filter11/1(F_Signal_out) -> L4 drop/1(Vabc_start)
  [V3] -> Filter8/1(Signal_in)
  [Milk_RP] -> Milk processing plant/2(Q)
  Solar supply power factor/1(pf) -> [INV_pf], Solar infeed pf/1  "Solar infeed pf"
  Milk machine profile/2 -> [Milk_RP]
  Filter7/1(F_Signal_out) -> Single phase _loads_ Loading/3(Iabc_out)
  [water_s] -> Water pump power factor/2(Total_S)
  [Milk_AP] -> Milk processing plant/1(P)
  [V3] -> Filter9/1(Signal_in)
  Water pump profile/2 -> [Water_RP]
  [Q3] -> Water pump output/2
  [Water_AP] -> Water Pump/1(P)
  [P3] -> Water pump power factor/1(Total_P)
  Maize mill profile/1 -> [Maize_AP]
  [T1_L] -> Bus Creator/1
  [T2_L] -> Bus Creator/2
  Bus Creator/1 -> Transformer _loading/1
  [INV_pf] -> Bus Creator1/1
  [INV_S] -> Bus Creator1/2
  Bus Creator1/1 -> Solar infeed parameters/1
  [Total_P] -> Bus Creator2/1
  [Total_Q] -> Bus Creator2/2
  [Total_S] -> Bus Creator2/3
  [sys_pf] -> Bus Creator2/4
  Bus Creator2/1 -> Feeder model parameters/1
  [Vdrop] -> Bus Creator3/1
  [Vdrop_L1] -> Bus Creator3/2
  [Vdrop_L2] -> Bus Creator3/3
  [Vdrop_L3] -> Bus Creator3/4
  [Vdrop_L4] -> Bus Creator3/5
  Bus Creator3/1 -> Feeder voltage drop data/1
  [INV_A] -> Bus Creator1/3
  Domestic loads/2 -> [Dom_RP]
  Domestic loads/1 -> [Dom_AP]
  Domestic /Residential loads(0.23kV)/2(Pout) -> [P4]
  Domestic /Residential loads(0.23kV)/3(Qout) -> [Q4]
  Domestic /Residential loads(0.23kV)/1(P_seq_v) -> Terminator3/1
  [Dom_RP] -> Domestic /Residential loads(0.23kV)/2(Q)
  [Dom_AP] -> Domestic /Residential loads(0.23kV)/1(P)
  [P4] -> Domestic_loads/1(P)
  [Q4] -> Domestic_loads/2(Q)
  [Q4] -> Domestic loads_output/2
  [P4] -> Domestic loads_output/1
  connections:
  Vin,Iin/RConn2 -- Three-Phase Source1/RConn2 -- V1,I1/LConn2 -- "11kV/400V "/RConn2
  V6,I6/RConn3 -- Domestic /Residential loads(0.23kV)/LConn3
  Vin,Iin/RConn3 -- Three-Phase Source1/RConn3 -- V1,I1/LConn3 -- "11kV/400V "/RConn3
  Milk processing plant/LConn2 -- "400/230V-10kVA "/LConn2 -- L3_5km/LConn2 -- V3,I3/RConn2
  Maize mill/LConn3 -- V2,I2/RConn3 -- L2_3km/LConn3
  "400/230V-10kVA "/LConn3 -- V3,I3/RConn3 -- L3_5km/LConn3 -- Milk processing plant/LConn3
  V6,I6/RConn2 -- Domestic /Residential loads(0.23kV)/LConn2
  Maize mill/LConn2 -- V2,I2/RConn2 -- L2_3km/LConn2
  Milk processing plant/LConn1 -- V3,I3/RConn1 -- "400/230V-10kVA "/LConn1 -- L3_5km/LConn1
  Vin,Iin/RConn1 -- Three-Phase Source1/RConn1 -- V1,I1/LConn1 -- "11kV/400V "/RConn1
  Maize mill/LConn1 -- V2,I2/RConn1 -- L2_3km/LConn1
  Domestic /Residential loads(0.23kV)/LConn1 -- V6,I6/RConn1
  L3_5km/RConn1 -- V4,I4/LConn1
  L4_5km/LConn3 -- V5,I5/RConn1
  V4,I4/RConn1 -- Water Pump/LConn1
  L4_5km/RConn3 -- V6,I6/LConn1
  V_Input_B/RConn1 -- Vin,Iin/LConn2
  "400/230V-10kVA "/RConn3 -- V5,I5/LConn3
  L1_10km/LConn3 -- V1,I1/RConn3
  V_Input_A/RConn1 -- Vin,Iin/LConn1
  L4_5km/RConn2 -- V6,I6/LConn2
  L1_10km/RConn3 -- V2,I2/LConn3
  L1_10km/RConn2 -- V2,I2/LConn2
  11kV Main supply/RConn1 -- "11kV/400V "/LConn1
  L4_5km/LConn1 -- V5,I5/RConn3
  L1_10km/RConn1 -- V2,I2/LConn1
  V5,I5/LConn1 -- "400/230V-10kVA "/RConn1
  V_Input_C/RConn1 -- Vin,Iin/LConn3
  11kV Main supply/RConn2 -- "11kV/400V "/LConn2
  L1_10km/LConn1 -- V1,I1/RConn1
  L3_5km/RConn2 -- V4,I4/LConn2
  L4_5km/RConn1 -- V6,I6/LConn3
  L4_5km/LConn2 -- V5,I5/RConn2
  L2_3km/RConn2 -- V3,I3/LConn2
  V5,I5/LConn2 -- "400/230V-10kVA "/RConn2
  11kV Main supply/RConn3 -- "11kV/400V "/LConn3
  L3_5km/RConn3 -- V4,I4/LConn3
  L1_10km/LConn2 -- V1,I1/RConn2
  V4,I4/RConn3 -- Water Pump/LConn3
  L2_3km/RConn3 -- V3,I3/LConn3
  L2_3km/RConn1 -- V3,I3/LConn1
  V4,I4/RConn2 -- Water Pump/LConn2

== system PV_&_LV_FEEDER_MODEL/Filter1 ==
  Signal_in : Inport
  First-Order Filter18 : spsFirstOrderFilterLib/First-Order Filter  FilterType=Lowpass  Tc=1/(2*pi*50)  Ts=0  Initialize=off  Vac_Init=[0, 0, 50]  Vdc_Init=0  PlotResponse=off  FreqRange="[0,  200,  1]"
  First-Order Filter19 : spsFirstOrderFilterLib/First-Order Filter  FilterType=Lowpass  Tc=1/(2*pi*50)  Ts=0  Initialize=off  Vac_Init=[0, 0, 50]  Vdc_Init=0  PlotResponse=off  FreqRange="[0,  200,  1]"
  First-Order Filter20 : spsFirstOrderFilterLib/First-Order Filter  FilterType=Lowpass  Tc=1/(2*pi*50)  Ts=0  Initialize=off  Vac_Init=[0, 0, 50]  Vdc_Init=0  PlotResponse=off  FreqRange="[0,  200,  1]"
  F_Signal_out : Outport
  wires:
  First-Order Filter18/1 -> First-Order Filter19/1
  First-Order Filter20/1 -> F_Signal_out/1
  First-Order Filter19/1 -> First-Order Filter20/1
  Signal_in/1 -> First-Order Filter18/1
